simulink model "APSensor"  (R2023a)
settings: Solver=VariableStepAuto  StartTime=0.0  StopTime=10.0  RelTol=1e-3
settings Model: Creator=Egypt_Laptop  LastModifiedBy=Egypt_Laptop

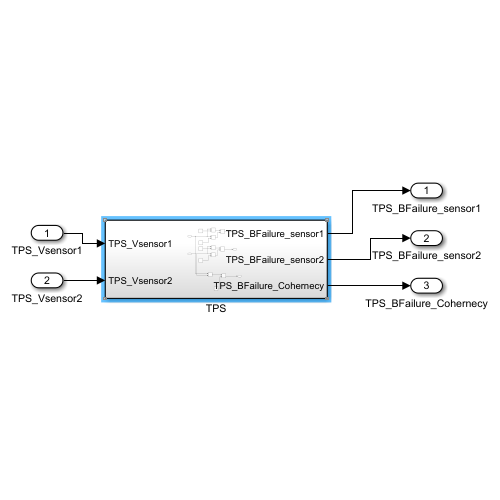
[thumbnail: Simulink's stored preview of the top-level diagram]
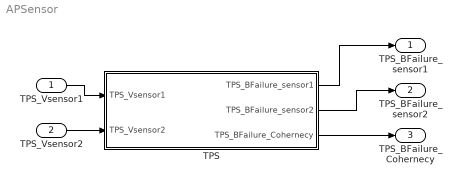
== system APSensor ==
  TPS_Vsensor1 : Inport  OutDataTypeStr=single
  TPS_Vsensor2 : Inport  Port=2  OutDataTypeStr=single
  TPS : Subsystem
  TPS_BFailure_sensor1 : Outport
  TPS_BFailure_sensor2 : Outport  Port=2
  TPS_BFailure_Cohernecy : Outport  Port=3
  wires:
  TPS/3(TPS_BFailure_Cohernecy) -> TPS_BFailure_Cohernecy/1
  TPS_Vsensor1/1 -> TPS/1(TPS_Vsensor1)
  TPS_Vsensor2/1 -> TPS/2(TPS_Vsensor2)
  TPS/2(TPS_BFailure_sensor2) -> TPS_BFailure_sensor2/1
  TPS/1(TPS_BFailure_sensor1) -> TPS_BFailure_sensor1/1

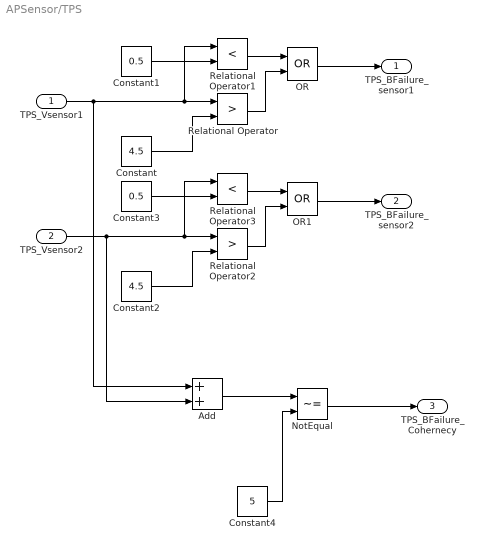
== system APSensor/TPS ==
  TPS_Vsensor1 : Inport  OutDataTypeStr=single
  TPS_Vsensor2 : Inport  Port=2  OutDataTypeStr=single
  Add : Sum
  Constant : Constant  Value=4.5
  Constant1 : Constant  Value=0.5
  Constant2 : Constant  Value=4.5
  Constant3 : Constant  Value=0.5
  Constant4 : Constant  Value=5
  NotEqual : RelationalOperator  Operator=~=  OutDataTypeStr=boolean  RndMeth=Simplest  InputSameDT=off
  OR : Logic  Operator=OR  AllPortsSameDT=off  OutDataTypeStr=boolean
  OR1 : Logic  Operator=OR  AllPortsSameDT=off  OutDataTypeStr=boolean
  Relational Operator : RelationalOperator  Operator=>  OutDataTypeStr=boolean  RndMeth=Simplest  InputSameDT=off
  Relational Operator1 : RelationalOperator  Operator=<  OutDataTypeStr=boolean  RndMeth=Simplest  InputSameDT=off
  Relational Operator2 : RelationalOperator  Operator=>  OutDataTypeStr=boolean  RndMeth=Simplest  InputSameDT=off
  Relational Operator3 : RelationalOperator  Operator=<  OutDataTypeStr=boolean  RndMeth=Simplest  InputSameDT=off
  TPS_BFailure_sensor1 : Outport  OutDataTypeStr=boolean
  TPS_BFailure_sensor2 : Outport  Port=2  OutDataTypeStr=boolean
  TPS_BFailure_Cohernecy : Outport  Port=3  OutDataTypeStr=boolean
  wires:
  Constant/1 -> Relational Operator/2
  Constant1/1 -> Relational Operator1/2
  OR1/1 -> TPS_BFailure_sensor2/1
  Constant2/1 -> Relational Operator2/2
  Constant3/1 -> Relational Operator3/2
  TPS_Vsensor1/1 -> Add/1, Relational Operator1/1, Relational Operator/1
  TPS_Vsensor2/1 -> Add/2, Relational Operator2/1, Relational Operator3/1
  Relational Operator/1 -> OR/2
  Relational Operator1/1 -> OR/1
  Relational Operator3/1 -> OR1/1
  Relational Operator2/1 -> OR1/2
  OR/1 -> TPS_BFailure_sensor1/1
  Add/1 -> NotEqual/1
  NotEqual/1 -> TPS_BFailure_Cohernecy/1
  Constant4/1 -> NotEqual/2
